simulink model "lab_3"  (R2021b)
settings: Solver=VariableStepAuto  StartTime=0.0  StopTime=t  MaxStep=1e-2  RelTol=1e-3
values from neighbouring files (symbols this model uses):
  a1 = 5    [script_lab_3.m]
  a2 = 1    [script_lab_3.m]
  direct = 0    [script_lab_3.m]
  K = acker(A,b,p)    [script_lab_3.m]
  kn = 1 / (-c/(A-b*K)*b)    [script_lab_3.m]
  L = acker(A',c',p)    [script_lab_3.m]
  observer = 1    [script_lab_3.m]
  x1_0 = i    [script_lab_3.m]
  x2_0 = i    [script_lab_3.m]
settings Model: Creator=79159  LastModifiedBy=79159

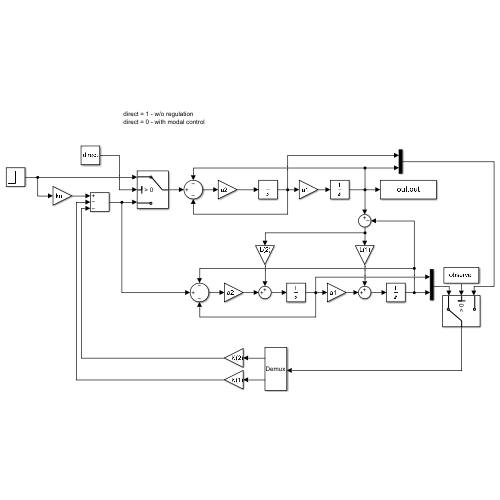
[thumbnail: Simulink's stored preview of the top-level diagram]
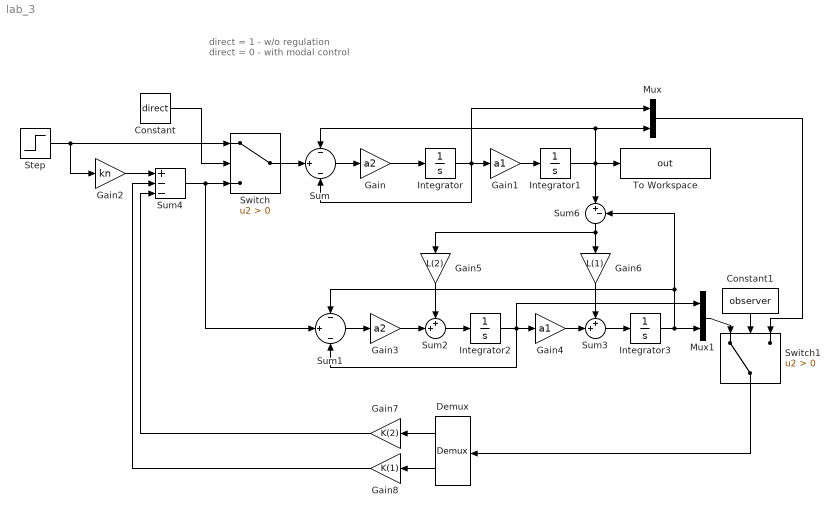
== system lab_3 ==
  note: direct = 1 - w/o regulation
      | direct = 0 - with modal control
  Constant : Constant  Value=direct
  Constant1 : Constant  Value=observer
  Demux : Demux  Outputs=2
      settings: DisplayOption=none
  Gain : Gain  Gain=a2
  Gain1 : Gain  Gain=a1
  Gain2 : Gain  Gain=kn
  Gain3 : Gain  Gain=a2
  Gain4 : Gain  Gain=a1
  Gain5 : Gain  Gain=L(2)
  Gain6 : Gain  Gain=L(1)
  Gain7 : Gain  Gain=K(2)
  Gain8 : Gain  Gain=K(1)
  Integrator : Integrator  InitialCondition=x1_0
  Integrator1 : Integrator  InitialCondition=x2_0
  Integrator2 : Integrator
  Integrator3 : Integrator
  Mux : Mux  Inputs=2
  Mux1 : Mux  Inputs=2
  Step : Step  Time=0  SampleTime=0
  Sum : Sum  Inputs=-|+|-
  Sum1 : Sum  Inputs=-|+|-
  Sum2 : Sum  Inputs=++|
  Sum3 : Sum  Inputs=++|
  Sum4 : Sum  Inputs=+--
  Sum6 : Sum  Inputs=|+-
  Switch : Switch  Criteria=u2 > Threshold
  Switch1 : Switch  Criteria=u2 > Threshold
  To Workspace : ToWorkspace  VariableName=out  SaveFormat=Timeseries  SampleTime=-1
  wires:
  Sum/1 -> Gain/1
  Gain/1 -> Integrator/1
  Gain1/1 -> Integrator1/1
  Integrator/1 -> Mux/1, Sum/3, Gain1/1
  Integrator1/1 -> Mux/2, Sum/1, Sum6/1, To Workspace/1
  Integrator3/1 -> Mux1/2, Sum6/2, Sum1/1
  Integrator2/1 -> Mux1/1, Gain4/1, Sum1/3
  Sum1/1 -> Gain3/1
  Gain3/1 -> Sum2/2
  Sum2/1 -> Integrator2/1
  Gain4/1 -> Sum3/2
  Sum3/1 -> Integrator3/1
  Gain5/1 -> Sum2/1
  Gain6/1 -> Sum3/1
  Gain7/1 -> Sum4/3
  Gain8/1 -> Sum4/2
  Sum6/1 -> Gain5/1, Gain6/1
  Constant/1 -> Switch/2
  Step/1 -> Gain2/1, Switch/1
  Switch/1 -> Sum/2
  Sum4/1 -> Switch/3, Sum1/2
  Gain2/1 -> Sum4/1
  Constant1/1 -> Switch1/2
  Mux/1 -> Switch1/3
  Switch1/1 -> Demux/1
  Demux/1 -> Gain7/1
  Demux/2 -> Gain8/1
  Mux1/1 -> Switch1/1
